simulink model "Problem_8_FlowChart"  (R2020a)
settings: Solver=VariableStepAuto  StartTime=0.0  StopTime=10.0  RelTol=1e-3
settings Model: Creator=Admin  LastModifiedBy=Admin

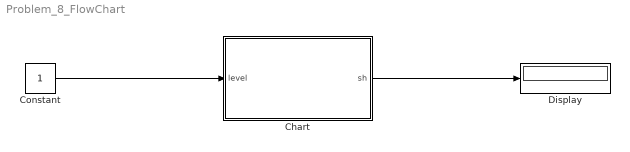
== system Problem_8_FlowChart ==
  Chart : Stateflow chart  TreatAsAtomicUnit=on
  Constant : Constant
  Display : Display
  wires:
  Constant/1 -> Chart/1(level)
  Chart/1(sh) -> Display/1

== stateflow chart Problem_8_FlowChart/Chart ==
  (default) -> (junction 1) : {cur_st=0;}
  (junction 5) -> (junction 1) [order 2] : [cur_st~=level]
  (junction 1) -> (junction 3) [order 1] : [cur_st<=level]
  (junction 1) -> (junction 6) [order 2]
  (junction 3) -> (junction 4) : {cur_st=cur_st+1;}
  (junction 6) -> (junction 7) [order 2] : [cur_st>=level]
  (junction 6) -> (junction 5) [order 1] : {cur_st=0;}
  (junction 7) -> (junction 8) : {cur_st=cur_st-1;}
  (junction 8) -> (junction 5)
  (junction 4) -> (junction 8)
  (junction 5) -> (junction 9) [order 1] : {sh=cur_st;}
  data: level input; sh output; cur_st local =0
